simulink model "Simulink_Model"  (R2016b)
settings: Solver=FixedStepDiscrete  StartTime=0.0  StopTime=3600  FixedStep=0.01  RelTol=1e-3
values from neighbouring files (symbols this model uses):
  C = 1000    [CONSTANTS.m]
  Cc = 9100    [CONSTANTS.m]
  Ccov = 0.6    [CONSTANTS.m]
  Ch = 9100    [CONSTANTS.m]
  CK = 2    [CONSTANTS.m]
  Cp = 718    [CONSTANTS.m]
  H = 1000    [CONSTANTS.m]
  H_const = 0.0    (= 0)    [CONSTANTS.m]
  Hcov = 0.7    [CONSTANTS.m]
  HK = 5    [CONSTANTS.m]
  HTC = 0.5    [CONSTANTS.m]
  Low_Target = 274    [CONSTANTS.m]
  mc = 0.113/2.45    (= 0.0461224489796)    [CONSTANTS.m]
  mh = 0.293/2    (= 0.1465)    [CONSTANTS.m]
  Qc = Cc * mc * T    (= 123396)    [CONSTANTS.m]    (also in heat_caps.m = 2*(To-Ti)/Rt; heat_caps2.m = (To-Ti)/Rt)
  Qh = Ch * mh * T    (= 391946.1)    [CONSTANTS.m]
  Qp = Cp*V*1.2754*T    (= 403.8401052)    [CONSTANTS.m]
  Rtc = 0.7    [CONSTANTS.m]
  Rth = 0.152    [CONSTANTS.m]
  Rtp = 6.25*0.8    (= 5)    [CONSTANTS.m]
  T = 294    [CONSTANTS.m]
  Up_Target = 276    [CONSTANTS.m]
  V = .0015    (= 0.0015)    [CONSTANTS.m]
undefined symbols (not defined in the file or in its folder): DiscIntNeverNeededParam
settings Model: NumberOfSteps=10  Creator=Evan  LastModifiedBy=Evan

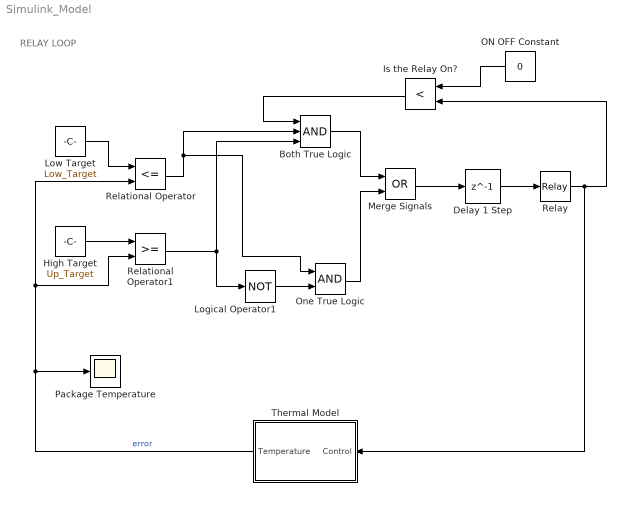
== system Simulink_Model ==
  note: RELAY
      | LOOP
  Both True Logic : Logic  Inputs=3  AllPortsSameDT=off  OutDataTypeStr=boolean
  Delay 1 Step : Delay  DelayLength=1
  High Target : Constant  Value=Up_Target
  Is the Relay On? : RelationalOperator  Operator=<  OutDataTypeStr=boolean  RndMeth=Simplest
  Logical Operator1 : Logic  Operator=NOT  AllPortsSameDT=off  OutDataTypeStr=boolean
  Low Target : Constant  Value=Low_Target
  Merge Signals : Logic  Operator=OR  AllPortsSameDT=off  OutDataTypeStr=boolean
  ON OFF Constant : Constant  Value=0
  One True Logic : Logic  AllPortsSameDT=off  OutDataTypeStr=boolean
  Package Temperature : Scope
  Relational Operator : RelationalOperator  Operator=<=  OutDataTypeStr=boolean  RndMeth=Simplest
  Relational Operator1 : RelationalOperator  OutDataTypeStr=boolean  RndMeth=Simplest
  Relay : Relay  OnOutputValue=Voltage  OutDataTypeStr=double
  Thermal Model : Subsystem
  wires:
  Thermal Model/1(Temperature) -> Package Temperature/1, Relational Operator1/2, Relational Operator/2  "error"
  Low Target/1 -> Relational Operator/1
  High Target/1 -> Relational Operator1/1
  Relational Operator1/1 -> Logical Operator1/1, Both True Logic/3
  Relational Operator/1 -> One True Logic/1, Both True Logic/2
  ON OFF Constant/1 -> Is the Relay On?/1
  Relay/1 -> Is the Relay On?/2, Thermal Model/1(Control)
  Merge Signals/1 -> Delay 1 Step/1
  Delay 1 Step/1 -> Relay/1
  Logical Operator1/1 -> One True Logic/2
  One True Logic/1 -> Merge Signals/2
  Is the Relay On?/1 -> Both True Logic/1
  Both True Logic/1 -> Merge Signals/1

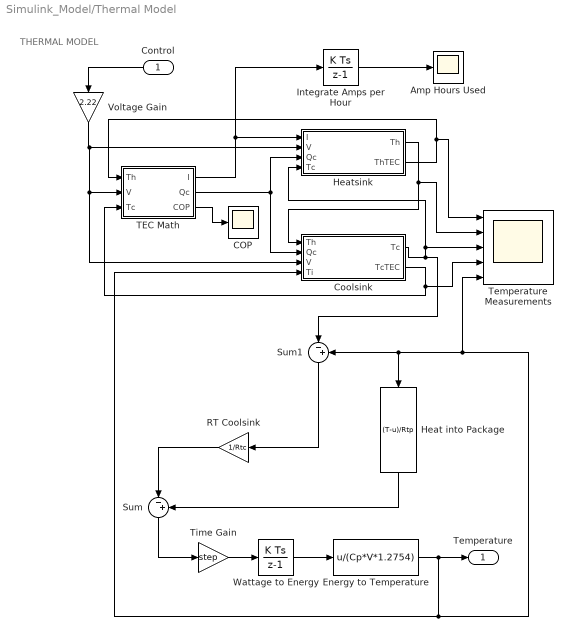
== system Simulink_Model/Thermal Model ==
  note: THERMAL
      | MODEL
  Control : Inport
  Amp Hours Used : Scope
  COP : Scope
  Coolsink : Subsystem
  Energy to Temperature : Fcn  Expr=u/(Cp*V*1.2754)
  Heat into Package : Fcn  Expr=(T-u)/Rtp
  Heatsink : Subsystem
  Integrate Amps per Hour : DiscreteIntegrator  gainval=1/(3600)*step  InitialConditionSetting=State (most efficient)  SampleTime=-1  ICPrevOutput=DiscIntNeverNeededParam  ICPrevScaledInput=DiscIntNeverNeededParam
  "RT Coolsink " : Gain  Gain=1/Rtc
  Sum : Sum  Inputs=|-+
  Sum1 : Sum  Inputs=|-+
  TEC Math : MATLAB Function  TreatAsAtomicUnit=on
  Temperature Measurements : Scope  NumInputPorts=5
  Time Gain : Gain  Gain=step
  Voltage Gain : Gain  Gain=2.22
  Wattage to Energy : DiscreteIntegrator  InitialCondition=Qp  InitialConditionSetting=State (most efficient)  SampleTime=-1  ICPrevOutput=DiscIntNeverNeededParam  ICPrevScaledInput=DiscIntNeverNeededParam
  Temperature : Outport
  wires:
  Control/1 -> Voltage Gain/1
  Voltage Gain/1 -> TEC Math/2(V), Coolsink/3(V), Heatsink/2(V)
  TEC Math/2(Qc) -> Heatsink/3(Qc), Coolsink/2(Qc)
  Heatsink/1(Th) -> Temperature Measurements/2, Coolsink/1(Th)
  TEC Math/1(I) -> Integrate Amps per Hour/1, Heatsink/1(I)
  Heat into Package/1 -> Sum/2
  Sum/1 -> Time Gain/1
  Time Gain/1 -> Wattage to Energy/1
  Wattage to Energy/1 -> Energy to Temperature/1
  Coolsink/1(Tc) -> Heatsink/4(Tc), Temperature Measurements/3, Sum1/1
  "RT Coolsink "/1 -> Sum/1
  Energy to Temperature/1 -> Temperature/1, Temperature Measurements/5, Sum1/2, Heat into Package/1, Coolsink/4(Ti)
  TEC Math/3(COP) -> COP/1
  Integrate Amps per Hour/1 -> Amp Hours Used/1
  Sum1/1 -> "RT Coolsink "/1
  Heatsink/2(ThTEC) -> Temperature Measurements/1, TEC Math/1(Th)
  Coolsink/2(TcTEC) -> Temperature Measurements/4, TEC Math/3(Tc)

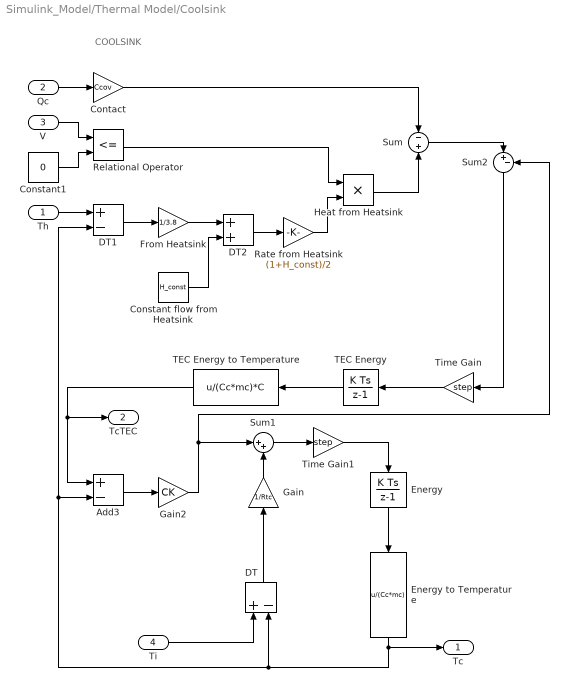
== system Simulink_Model/Thermal Model/Coolsink ==
  note: COOLSINK
  Th : Inport
  Qc : Inport  Port=2
  V : Inport  Port=3
  Ti : Inport  Port=4
  Add3 : Sum  Inputs=+-
  Constant flow from Heatsink : Constant  Value=H_const
  Constant1 : Constant  Value=0
  Contact : Gain  Gain=Ccov
  DT : Sum  Inputs=+-
  DT1 : Sum  Inputs=+-
  DT2 : Sum
  Energy : DiscreteIntegrator  InitialCondition=Qc  InitialConditionSetting=State (most efficient)  SampleTime=-1  ICPrevOutput=DiscIntNeverNeededParam  ICPrevScaledInput=DiscIntNeverNeededParam
  Energy to Temperature : Fcn  Expr=u/(Cc*mc)
  From Heatsink : Gain  Gain=1/3.8
  Gain : Gain  Gain=1/Rtc
  Gain2 : Gain  Gain=CK
  Heat from Heatsink : Product
  Rate from Heatsink : Gain  Gain=(1+H_const)/2
  Relational Operator : RelationalOperator  Operator=<=  OutDataTypeStr=boolean  RndMeth=Simplest
  Sum : Sum  Inputs=-+
  Sum1 : Sum  Inputs=|++
  Sum2 : Sum  Inputs=|+-
  TEC Energy : DiscreteIntegrator  InitialCondition=Qc/C  InitialConditionSetting=State (most efficient)  SampleTime=-1  ICPrevOutput=DiscIntNeverNeededParam  ICPrevScaledInput=DiscIntNeverNeededParam
  TEC Energy to Temperature : Fcn  Expr=u/(Cc*mc)*C
  Time Gain : Gain  Gain=step
  Time Gain1 : Gain  Gain=step
  Tc : Outport
  TcTEC : Outport  Port=2
  wires:
  Energy/1 -> Energy to Temperature/1
  Qc/1 -> Contact/1
  Contact/1 -> Sum/1
  DT/1 -> Gain/1
  Gain/1 -> Sum1/2
  Th/1 -> DT1/1
  DT1/1 -> From Heatsink/1
  Constant1/1 -> Relational Operator/2
  Heat from Heatsink/1 -> Sum/2
  V/1 -> Relational Operator/1
  Relational Operator/1 -> Heat from Heatsink/1
  DT2/1 -> Rate from Heatsink/1
  From Heatsink/1 -> DT2/1
  Rate from Heatsink/1 -> Heat from Heatsink/2
  Constant flow from Heatsink/1 -> DT2/2
  TEC Energy/1 -> TEC Energy to Temperature/1
  Ti/1 -> DT/1
  TEC Energy to Temperature/1 -> Add3/1, TcTEC/1
  Energy to Temperature/1 -> Tc/1, Add3/2, DT1/2, DT/2
  Sum2/1 -> Time Gain/1
  Gain2/1 -> Sum1/1, Sum2/2
  Add3/1 -> Gain2/1
  Sum/1 -> Sum2/1
  Sum1/1 -> Time Gain1/1
  Time Gain/1 -> TEC Energy/1
  Time Gain1/1 -> Energy/1

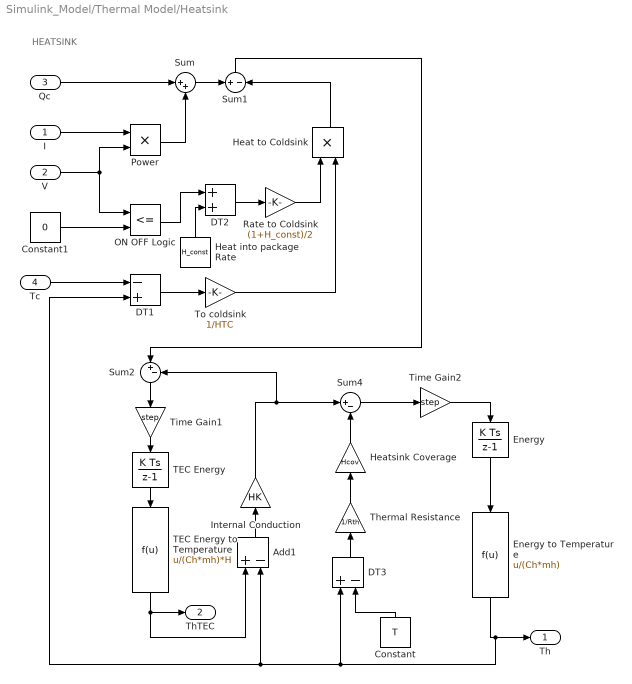
== system Simulink_Model/Thermal Model/Heatsink ==
  note: HEATSINK
  I : Inport
  V : Inport  Port=2
  Qc : Inport  Port=3
  Tc : Inport  Port=4
  Add1 : Sum  Inputs=+-
  Constant : Constant  Value=T
  Constant1 : Constant  Value=0
  DT1 : Sum  Inputs=-+
  DT2 : Sum
  DT3 : Sum  Inputs=+-
  Energy : DiscreteIntegrator  InitialCondition=Qh  InitialConditionSetting=State (most efficient)  SampleTime=-1  ICPrevOutput=DiscIntNeverNeededParam  ICPrevScaledInput=DiscIntNeverNeededParam
  Energy to Temperature : Fcn  Expr=u/(Ch*mh)
  Heat into package Rate : Constant  Value=H_const
  Heat to Coldsink : Product
  Heatsink Coverage : Gain  Gain=Hcov
  Internal Conduction : Gain  Gain=HK
  ON OFF Logic : RelationalOperator  Operator=<=  OutDataTypeStr=boolean  RndMeth=Simplest
  Power : Product
  Rate to Coldsink : Gain  Gain=(1+H_const)/2
  Sum : Sum  Inputs=|++
  Sum1 : Sum  Inputs=+-
  Sum2 : Sum  Inputs=|+-
  Sum4 : Sum  Inputs=|+-
  TEC Energy : DiscreteIntegrator  InitialCondition=Qh/H  InitialConditionSetting=State (most efficient)  SampleTime=-1  ICPrevOutput=DiscIntNeverNeededParam  ICPrevScaledInput=DiscIntNeverNeededParam
  TEC Energy to Temperature : Fcn  Expr=u/(Ch*mh)*H
  Thermal Resistance : Gain  Gain=1/Rth
  Time Gain1 : Gain  Gain=step
  Time Gain2 : Gain  Gain=step
  To coldsink : Gain  Gain=1/HTC
  Th : Outport
  ThTEC : Outport  Port=2
  wires:
  Qc/1 -> Sum/1
  Power/1 -> Sum/2
  V/1 -> ON OFF Logic/1, Power/2
  Energy/1 -> Energy to Temperature/1
  I/1 -> Power/1
  DT1/1 -> To coldsink/1
  Tc/1 -> DT1/1
  Sum/1 -> Sum1/1
  Constant1/1 -> ON OFF Logic/2
  To coldsink/1 -> Heat to Coldsink/2
  Heat to Coldsink/1 -> Sum1/2
  ON OFF Logic/1 -> DT2/1
  Heat into package Rate/1 -> DT2/2
  DT2/1 -> Rate to Coldsink/1
  Rate to Coldsink/1 -> Heat to Coldsink/1
  TEC Energy/1 -> TEC Energy to Temperature/1
  TEC Energy to Temperature/1 -> Add1/1, ThTEC/1
  Add1/1 -> Internal Conduction/1
  Internal Conduction/1 -> Sum4/1, Sum2/2
  Sum1/1 -> Sum2/1
  Heatsink Coverage/1 -> Sum4/2
  DT3/1 -> Thermal Resistance/1
  Energy to Temperature/1 -> DT3/1, DT1/2, Add1/2, Th/1
  Constant/1 -> DT3/2
  Thermal Resistance/1 -> Heatsink Coverage/1
  Sum4/1 -> Time Gain2/1
  Sum2/1 -> Time Gain1/1
  Time Gain1/1 -> TEC Energy/1
  Time Gain2/1 -> Energy/1

== matlab function Simulink_Model/Thermal Model/TEC Math ==
  data: Th input; I output; V input; Tc input; Qc output; COP output
function [I, Qc, COP] = fcn(Th, V, Tc)
%{
TEC Math
This function runs TEC math to get the current draw, the heat transfer
rate, and the coefficient of performance.

Parameters: temperature hot side, voltage, temperature cold side

Returns: current, heat transfer rate, coefficient of performance

Evan Bosia
%}

n = 127;    %number of TEC couples in new TEC
Inew = 4.8; %Imax of new TEC

%Constants for TEC with 71 couples and Imax of 6 amps
s1 = 1.33450 * 10^-2; 
s2 = -5.37574 * 10^-5; 
s3 = 7.42731 * 10^-7;
s4 = -1.27141 * 10^-9;

r1 = 2.08317; 
r2 = -1.98763 * 10^-2; 
r3 = 8.53832 * 10^-5; 
r4 = -9.03143 * 10^-8;

k1 = 4.76218 * 10^-1;
k2 = -3.89821 * 10^-6;
k3 = -8.64864 * 10^-6;
k4 = 2.20869 * 10^-8;

%Temperature difference between hot and cold side
DT = (Th-Tc);

%Equations dependent on temperature difference
if(DT == 0)
    T = Th;
    Sm = s1 + s2*T + s3*T^2 + s4*T^3;
    Rm = r1 + r2*T + r3*T^2 + r4*T^3;
    Km = k1 + k2*T + k3*T^2 + k4*T^3;
else
    Smh = s1*Th + (s2*Th^2)/2 + (s3*Th^3)/3 + (s4*Th^4)/4;
    Smc = s1*Tc + (s2*Tc^2)/2 + (s3*Tc^3)/3 + (s4*Tc^4)/4;
    Sm = (Smh - Smc)/DT;

    Rmh = r1*Th + (r2*Th^2)/2 + (r3*Th^3)/3 + (r4*Th^4)/4;
    Rmc = r1*Tc + (r2*Tc^2)/2 + (r3*Tc^3)/3 + (r4*Tc^4)/4;
    Rm = (Rmh - Rmc)/DT;

    Kmh = k1*Th + (k2*Th^2)/2 + (k3*Th^3)/3 + (k4*Th^4)/4;
    Kmc = k1*Tc + (k2*Tc^2)/2 + (k3*Tc^3)/3 + (k4*Tc^4)/4;
    Km = (Kmh - Kmc)/DT;
end

%Convert to new TEC
Sm = Sm * (n/71);
Rm = Rm * (n/71) * (6/Inew);
Km = Km * (n/71) * (Inew/6);

%Current
I = (V - (Sm * DT))/Rm;

%Heat transfer rate
Qc = ((Sm * Tc * I) - (0.5 * I^2 * Rm) - (Km * DT));

%Power
P = I*V;

%If the current is negative, set power to a high value
if(P <= 0)
   P = 1000000; 
end

%If the TEC is unpowered, set Qc to the -temperature differential * Rt, I
%to 0 and COP to 0
if(V <= 0)
    Qc = -DT/1.6;
    I = 0;
    COP = 0;
else
    COP = Qc / P;
end

end
